simulink model "test_direct"  (R2024a)
settings: Solver=VariableStepAuto  StartTime=0.0  StopTime=40  RelTol=1e-3
libraries: neural x733, simulink x4
(part 16 of 35)

== system test_direct/Function Fitting Neural Network2/Layer 4/Delays 1 ==
  "p{4}" : Inport  PortDimensions=20
      mask Display: e = 0.06;c1 = [120 230 180]/255;c2 = ([120 230 180]+0)/(256+128);c3 = ([120 230 180]+128)/(256+128);patch([0 1 1 0],[0 0 1 1],c1);patch([0 1 1 1-e 1-e 0+e],[0 0 1 1-e 0+e 0+e],c2);patch([0 0 1 1-e 0+e 0+e],[0 1 1 1-e 1-e 0+e],c3);plot([0 1 1 0 0],[0 0 1 1 0]);
  mux : Mux  Inputs=1
      mask Display: e = 0.06;c1 = [120 150 230]/255;c2 = ([120 150 230]+0)/383;c3 = ([120 150 230]+128)/383;patch([0 1 1 0],[0 0 1 1],c1);patch([0 1 1 1-e 1-e 0+e],[0 0 1 1-e 0+e 0+e],c2);patch([0 0 1 1-e 0+e 0+e],[0 1 1 1-e 1-e 0+e],c3);plot([0 1 1 0 0],[0 0 1 1 0]);disp('Mux')
  "pd{4,3}" : Outport
      mask Display: e = 0.06;c1 = [120 230 180]/255;c2 = ([120 230 180]+0)/(256+128);c3 = ([120 230 180]+128)/(256+128);patch([0 1 1 0],[0 0 1 1],c1);patch([0 1 1 1-e 1-e 0+e],[0 0 1 1-e 0+e 0+e],c2);patch([0 0 1 1-e 0+e 0+e],[0 1 1 1-e 1-e 0+e],c3);plot([0 1 1 0 0],[0 0 1 1 0]);
  wires:
  "p{4}"/1 -> mux/1
  mux/1 -> "pd{4,3}"/1

== system test_direct/Function Fitting Neural Network2/Layer 4/LW{4,3} ==
  "ad{4,3}" : Inport  PortDimensions=20
      mask Display: e = 0.06;c1 = [120 230 180]/255;c2 = ([120 230 180]+0)/(256+128);c3 = ([120 230 180]+128)/(256+128);patch([0 1 1 0],[0 0 1 1],c1);patch([0 1 1 1-e 1-e 0+e],[0 0 1 1-e 0+e 0+e],c2);patch([0 0 1 1-e 0+e 0+e],[0 1 1 1-e 1-e 0+e],c3);plot([0 1 1 0 0],[0 0 1 1 0]);
  "IW{4,3}(1,:)'" : Constant  Value=[0.47244748817045678634940486517734825611114501953125;0.1834479136632027607145545289313304238021373748779296875;0.50676050579155818009979839189327321946620941162109375;-0.319327133366968662908647047515842132270336151123046875;0.381766967450572980435907766150194220244884490966796875;0.4563690535882181098514820405398495495319366455078125;0.198247183159460271806295850183232687413692474365234375;-0.33336007021097657787578327770461328327655792236328125;-0.412713567221942578822080349709722213447093963623046875;0.450498773156788934191041562371538020670413970947265625;0.25918714352219252017306416746578179299831390380859375;0.410400201848454049269321330939419567584991455078125;0.5409615578128141866187661435105837881565093994140625;-0.1653232740233982200894757852438488043844699859619140625;-0.462903675222519073173543802113272249698638916015625;-0.291527346498789807771601090280455537140369415283203125;0.0824641426334296323563677333368104882538318634033203125;0.1511362276477953570097412239192635752260684967041015625;0.211910610504960905675631011035875417292118072509765625;0.2073592739845122323583126444646040908992290496826171875]
      mask Display: e = 0.06;c1 = [120 150 230]/255;c2 = ([120 150 230]+0)/383;c3 = ([120 150 230]+128)/383;patch([0 1 1 0],[0 0 1 1],c1);patch([0 1 1 1-e 1-e 0+e],[0 0 1 1-e 0+e 0+e],c2);patch([0 0 1 1-e 0+e 0+e],[0 1 1 1-e 1-e 0+e],c3);plot([0 1 1 0 0],[0 0 1 1 0]);disp('weights');
  "IW{4,3}(10,:)'" : Constant  Value=[0.62004982880781611687126542165060527622699737548828125;-0.1719950517254123789623321272301836870610713958740234375;-0.181893759276586075568360456600203178822994232177734375;-0.2349075039028051536948993316400446929037570953369140625;-0.2452130522313871463513379467258346267044544219970703125;0.53580241435795894489046986564062535762786865234375;0.1931726513438345171902454922019387595355510711669921875;0.416953523146994131653997328612604178488254547119140625;0.397838857842025495070714669054723344743251800537109375;0.507717044004438289306335718720220029354095458984375;-0.09416114315560132619342681437046849168837070465087890625;-0.041804193884274531978206823623622767627239227294921875;0.220907364886507029400064539004233665764331817626953125;-0.39379811215660531775739627846633084118366241455078125;0.022802943761242200348959840994211845099925994873046875;-0.1133939581571223043088281201562494970858097076416015625;-0.11496157101289783408759603844373486936092376708984375;0.43779622024544206926321976425242610275745391845703125;0.55289807234135668334573665561038069427013397216796875;-0.064019714526170112822711644184892065823078155517578125]
      mask Display: e = 0.06;c1 = [120 150 230]/255;c2 = ([120 150 230]+0)/383;c3 = ([120 150 230]+128)/383;patch([0 1 1 0],[0 0 1 1],c1);patch([0 1 1 1-e 1-e 0+e],[0 0 1 1-e 0+e 0+e],c2);patch([0 0 1 1-e 0+e 0+e],[0 1 1 1-e 1-e 0+e],c3);plot([0 1 1 0 0],[0 0 1 1 0]);disp('weights');
  "IW{4,3}(2,:)'" : Constant  Value=[-0.52999007124834929260970284303766675293445587158203125;0.25866553837085659584005270517081953585147857666015625;-0.480994413539897192055860841719550080597400665283203125;0.5206363297816836155362807403434999287128448486328125;-0.051047340005507368942971879732795059680938720703125;0.397809270661283853609546667939866892993450164794921875;0.3484531918175519660252348330686800181865692138671875;0.108374910894089293567077447733026929199695587158203125;-0.28461804870320717153475698069087229669094085693359375;0.39361667333479866126566548700793646275997161865234375;0.5237614091308453456719007590436376631259918212890625;-0.157341307151045384227217027728329412639141082763671875;0.2175219008468349812801534426398575305938720703125;-0.09173383416637879983479564316439791582524776458740234375;-0.57629988642295171263896236268919892609119415283203125;0.4459283104025819621796244973666034638881683349609375;0.2831475555888369743939847467117942869663238525390625;-0.342059279452377740238233627678710035979747772216796875;-0.17909678064247780415740862736129201948642730712890625;-0.1831357131080906530673502174977329559624195098876953125]
      mask Display: e = 0.06;c1 = [120 150 230]/255;c2 = ([120 150 230]+0)/383;c3 = ([120 150 230]+128)/383;patch([0 1 1 0],[0 0 1 1],c1);patch([0 1 1 1-e 1-e 0+e],[0 0 1 1-e 0+e 0+e],c2);patch([0 0 1 1-e 0+e 0+e],[0 1 1 1-e 1-e 0+e],c3);plot([0 1 1 0 0],[0 0 1 1 0]);disp('weights');
  "IW{4,3}(3,:)'" : Constant  Value=[0.427271557113994393528599857745575718581676483154296875;-0.2427281184362371779794642634442425332963466644287109375;0.375438812590348280906482614227570593357086181640625;0.1887302950483509267343151805107481777667999267578125;0.442888527891407146608315770208719186484813690185546875;-0.145704452211226131996824051384464837610721588134765625;0.19332090468647444847505312282009981572628021240234375;0.2171117569728686635954773009871132671833038330078125;-0.42483570338458431780992441417765803635120391845703125;0.416898792982427546238710647230618633329868316650390625;0.09328037965492620708918281025034957565367221832275390625;-0.297160611411257435943156224311678670346736907958984375;-0.222561662706281693235865759561420418322086334228515625;-0.63635994313177512982093730897759087383747100830078125;0.0920557715904673223850096519527141936123371124267578125;0.046618920974470602625050474898671382106840610504150390625;0.517752265816589396507652054424397647380828857421875;0.481589341247303848181360308444709517061710357666015625;0.50223095070663681394051991446758620440959930419921875;0.351524225397905787371399810581351630389690399169921875]
      mask Display: e = 0.06;c1 = [120 150 230]/255;c2 = ([120 150 230]+0)/383;c3 = ([120 150 230]+128)/383;patch([0 1 1 0],[0 0 1 1],c1);patch([0 1 1 1-e 1-e 0+e],[0 0 1 1-e 0+e 0+e],c2);patch([0 0 1 1-e 0+e 0+e],[0 1 1 1-e 1-e 0+e],c3);plot([0 1 1 0 0],[0 0 1 1 0]);disp('weights');
  "IW{4,3}(4,:)'" : Constant  Value=[-0.4272419811355068208769125703838653862476348876953125;-0.218328695116062287961966603688779287040233612060546875;-0.267850284719499065477776866828207857906818389892578125;0.06203137737339370350042599966400302946567535400390625;-0.55900733287565085305459433584474027156829833984375;0.2032377842318154603784563505541882477700710296630859375;-0.20301371483371821735630646799108944833278656005859375;0.2093600985184538298966572256176732480525970458984375;0.35642519122358684580120780083234421908855438232421875;-0.449654061964883833280026692591491155326366424560546875;-0.39742954838629085401180418557487428188323974609375;-0.376347479489261782514830656509730033576488494873046875;0.10974448386632405794127720355390920303761959075927734375;0.341992937278279451884799300387385301291942596435546875;0.422196331780901046304421697641373611986637115478515625;0.3298742516092314502884619287215173244476318359375;0.3378712155354772761484127840958535671234130859375;0.20815576754154696548226866070763207972049713134765625;0.357266630131023277261448356512119062244892120361328125;-0.344625803699752264463995743426494300365447998046875]
      mask Display: e = 0.06;c1 = [120 150 230]/255;c2 = ([120 150 230]+0)/383;c3 = ([120 150 230]+128)/383;patch([0 1 1 0],[0 0 1 1],c1);patch([0 1 1 1-e 1-e 0+e],[0 0 1 1-e 0+e 0+e],c2);patch([0 0 1 1-e 0+e 0+e],[0 1 1 1-e 1-e 0+e],c3);plot([0 1 1 0 0],[0 0 1 1 0]);disp('weights');
  "IW{4,3}(5,:)'" : Constant  Value=[0.242125074488241442960401172967976890504360198974609375;-0.60473759647022851115849562120274640619754791259765625;0.404473610734588817638979207913507707417011260986328125;-0.2590760492587571572897786609246395528316497802734375;0.1405439339409519095003275879207649268209934234619140625;0.142911761057261277318986003592726774513721466064453125;0.351091239707742974740511954223620705306529998779296875;0.0960644091923418541600909748012782074511051177978515625;-0.45544304543415237152004237941582687199115753173828125;-0.60626839080967542816580362341483123600482940673828125;0.42183625826601645059099610080011188983917236328125;-0.386967076793109321375396802977775223553180694580078125;-0.340070110055025021100760795889073051512241363525390625;0.1002300444043862370779862658309866674244403839111328125;-0.10990293007616182274777116845143609680235385894775390625;0.55207704769645282727452695326064713299274444580078125;-0.31459192782915545993915884537273086607456207275390625;0.345382987134464414236134643942932598292827606201171875;0.249144363683819924926154953936929814517498016357421875;0.168080126592327683265892801500740461051464080810546875]
      mask Display: e = 0.06;c1 = [120 150 230]/255;c2 = ([120 150 230]+0)/383;c3 = ([120 150 230]+128)/383;patch([0 1 1 0],[0 0 1 1],c1);patch([0 1 1 1-e 1-e 0+e],[0 0 1 1-e 0+e 0+e],c2);patch([0 0 1 1-e 0+e 0+e],[0 1 1 1-e 1-e 0+e],c3);plot([0 1 1 0 0],[0 0 1 1 0]);disp('weights');
  "IW{4,3}(6,:)'" : Constant  Value=[0.436176279970378499850625075850985012948513031005859375;-0.451489036951920663653936571790836751461029052734375;0.08911938882860499788751695859900792129337787628173828125;-0.485863711992422453445072960676043294370174407958984375;0.127572397355813327290974257266498170793056488037109375;-0.63812853495278332172091495522181503474712371826171875;0.2818837491960926033840451054857112467288970947265625;-0.0131968716074592172515789201270308694802224636077880859375;0.1537834832577880395110270228542503900825977325439453125;0.48011264273196319063430337337194941937923431396484375;-0.207405778126915352199688413747935555875301361083984375;-0.09951366702140125586328878171116230078041553497314453125;-0.268246262611988417479125246245530433952808380126953125;-0.406874531488279178592648577250656671822071075439453125;0.03159486549302327473842666449854732491075992584228515625;0.30773203396346981985942647952469997107982635498046875;0.033399545565028616878056055838897009380161762237548828125;-0.101874376296882063197557499734102748334407806396484375;0.048492904628586297466341648032539524137973785400390625;-0.34122312837322377188087330068810842931270599365234375]
      mask Display: e = 0.06;c1 = [120 150 230]/255;c2 = ([120 150 230]+0)/383;c3 = ([120 150 230]+128)/383;patch([0 1 1 0],[0 0 1 1],c1);patch([0 1 1 1-e 1-e 0+e],[0 0 1 1-e 0+e 0+e],c2);patch([0 0 1 1-e 0+e 0+e],[0 1 1 1-e 1-e 0+e],c3);plot([0 1 1 0 0],[0 0 1 1 0]);disp('weights');
  "IW{4,3}(7,:)'" : Constant  Value=[-0.283546119620839309760640389868058264255523681640625;-0.10361342455437162757281299718670197762548923492431640625;-0.058161527580973100548522580766075407154858112335205078125;0.51121075013165506728540776748559437692165374755859375;0.29651416162894383976578183137462474405765533447265625;-0.1252198113694278358565270536928437650203704833984375;-0.157886646248348305743292030456359498202800750732421875;0.32110978088458230761403910946683026850223541259765625;0.308480031707026258747106339797028340399265289306640625;0.033278433162800026556826793466825620271265506744384765625;0.396616284348000502912867659688345156610012054443359375;0.34965408898041838714476625682436861097812652587890625;0.326379064754532766112760100440937094390392303466796875;-0.26442051443391767495683097877190448343753814697265625;-0.325375298162383697064825582856428809463977813720703125;-0.17882765495459873594796817997121252119541168212890625;0.6391344025452669885822842843481339514255523681640625;0.66604526975968758595314511694596149027347564697265625;-0.5674698696229978356342371625942178070545196533203125;-0.0895385469065017314260757075317087583243846893310546875]
      mask Display: e = 0.06;c1 = [120 150 230]/255;c2 = ([120 150 230]+0)/383;c3 = ([120 150 230]+128)/383;patch([0 1 1 0],[0 0 1 1],c1);patch([0 1 1 1-e 1-e 0+e],[0 0 1 1-e 0+e 0+e],c2);patch([0 0 1 1-e 0+e 0+e],[0 1 1 1-e 1-e 0+e],c3);plot([0 1 1 0 0],[0 0 1 1 0]);disp('weights');
  "IW{4,3}(8,:)'" : Constant  Value=[-0.44158180291790649629746212667669169604778289794921875;-0.29737887161936871205369925519335083663463592529296875;-0.1731668100134340360085616339347325265407562255859375;-0.189524413062696350795732769256574101746082305908203125;-0.1682336544676640566198244641782366670668125152587890625;-0.63990017329392590017533848367747850716114044189453125;-0.12091324308068292225915030257965554483234882354736328125;-0.08116268648245718309031104809037060476839542388916015625;-0.1777960634037018816666630982581409625709056854248046875;-0.16733851128191801205247202233294956386089324951171875;0.489923677023728687540682358303456567227840423583984375;0.369528344926653040669606298251892440021038055419921875;-0.268289530246816509961860219846130348742008209228515625;-0.287624994977375647575712491743615828454494476318359375;0.17883429478338219720257029621279798448085784912109375;-0.48206985790917233902774796661105938255786895751953125;-0.009881485170639754678223454220642452128231525421142578125;0.448369826626772771671625150702311657369136810302734375;0.6902728087614977692254569774377159774303436279296875;0.354051711308562111479858458551461808383464813232421875]
      mask Display: e = 0.06;c1 = [120 150 230]/255;c2 = ([120 150 230]+0)/383;c3 = ([120 150 230]+128)/383;patch([0 1 1 0],[0 0 1 1],c1);patch([0 1 1 1-e 1-e 0+e],[0 0 1 1-e 0+e 0+e],c2);patch([0 0 1 1-e 0+e 0+e],[0 1 1 1-e 1-e 0+e],c3);plot([0 1 1 0 0],[0 0 1 1 0]);disp('weights');
  "IW{4,3}(9,:)'" : Constant  Value=[-0.471070051569210723751979230655706487596035003662109375;0.00431051595087869783562428693812762503512203693389892578125;-0.1575641998254519726696543102661962620913982391357421875;-0.072561288605265616968864605951239354908466339111328125;-0.5805348839554176354482706301496364176273345947265625;0.379023161422289034394594864352256990969181060791015625;-0.456586292726742615233348487890907563269138336181640625;-0.17056625130829339287430457261507399380207061767578125;0.24047114638423916499476717945071868598461151123046875;-0.1748905466580590317704491098993457853794097900390625;0.050215249866397672351414627200938411988317966461181640625;0.238950903829427574454058458286453969776630401611328125;-0.11299356269503146865673670617979951202869415283203125;-0.59749277719319981994061663499451242387294769287109375;-0.382383860884375759159325980363064445555210113525390625;-0.58043042099357389229652426365646533668041229248046875;-0.05488111243213793233319819364623981527984142303466796875;-0.49967492911579303171976107478258199989795684814453125;0.40333471589349245700617530019371770322322845458984375;0.31340698801696564856911209062673151493072509765625]
      mask Display: e = 0.06;c1 = [120 150 230]/255;c2 = ([120 150 230]+0)/383;c3 = ([120 150 230]+128)/383;patch([0 1 1 0],[0 0 1 1],c1);patch([0 1 1 1-e 1-e 0+e],[0 0 1 1-e 0+e 0+e],c2);patch([0 0 1 1-e 0+e 0+e],[0 1 1 1-e 1-e 0+e],c3);plot([0 1 1 0 0],[0 0 1 1 0]);disp('weights');
  Mux : Mux  Inputs=10
      mask Display: e = 0.06;c1 = [120 150 230]/255;c2 = ([120 150 230]+0)/383;c3 = ([120 150 230]+128)/383;patch([0 1 1 0],[0 0 1 1],c1);patch([0 1 1 1-e 1-e 0+e],[0 0 1 1-e 0+e 0+e],c2);patch([0 0 1 1-e 0+e 0+e],[0 1 1 1-e 1-e 0+e],c3);plot([0 1 1 0 0],[0 0 1 1 0]);disp('Mux');
  dotprod{1..10} (10 alike) : neural/Weight Functions/dotprod
  "lz{4,3}" : Outport
      mask Display: e = 0.06;c1 = [120 230 180]/255;c2 = ([120 230 180]+0)/(256+128);c3 = ([120 230 180]+128)/(256+128);patch([0 1 1 0],[0 0 1 1],c1);patch([0 1 1 1-e 1-e 0+e],[0 0 1 1-e 0+e 0+e],c2);patch([0 0 1 1-e 0+e 0+e],[0 1 1 1-e 1-e 0+e],c3);plot([0 1 1 0 0],[0 0 1 1 0]);
  wires:
  "IW{4,3}(1,:)'"/1 -> dotprod1/1
  "ad{4,3}"/1 -> dotprod1/2, dotprod2/2, dotprod3/2, dotprod4/2, dotprod5/2, dotprod6/2, dotprod7/2, dotprod8/2, dotprod9/2, dotprod10/2
  dotprod1/1 -> Mux/1
  "IW{4,3}(2,:)'"/1 -> dotprod2/1
  dotprod2/1 -> Mux/2
  "IW{4,3}(3,:)'"/1 -> dotprod3/1
  dotprod3/1 -> Mux/3
  "IW{4,3}(4,:)'"/1 -> dotprod4/1
  dotprod4/1 -> Mux/4
  "IW{4,3}(5,:)'"/1 -> dotprod5/1
  dotprod5/1 -> Mux/5
  "IW{4,3}(6,:)'"/1 -> dotprod6/1
  dotprod6/1 -> Mux/6
  "IW{4,3}(7,:)'"/1 -> dotprod7/1
  dotprod7/1 -> Mux/7
  "IW{4,3}(8,:)'"/1 -> dotprod8/1
  dotprod8/1 -> Mux/8
  "IW{4,3}(9,:)'"/1 -> dotprod9/1
  dotprod9/1 -> Mux/9
  "IW{4,3}(10,:)'"/1 -> dotprod10/1
  dotprod10/1 -> Mux/10
  Mux/1 -> "lz{4,3}"/1

== system test_direct/Function Fitting Neural Network2/Layer 5/Delays 1 ==
  "p{5}" : Inport  PortDimensions=10
      mask Display: e = 0.06;c1 = [120 230 180]/255;c2 = ([120 230 180]+0)/(256+128);c3 = ([120 230 180]+128)/(256+128);patch([0 1 1 0],[0 0 1 1],c1);patch([0 1 1 1-e 1-e 0+e],[0 0 1 1-e 0+e 0+e],c2);patch([0 0 1 1-e 0+e 0+e],[0 1 1 1-e 1-e 0+e],c3);plot([0 1 1 0 0],[0 0 1 1 0]);
  mux : Mux  Inputs=1
      mask Display: e = 0.06;c1 = [120 150 230]/255;c2 = ([120 150 230]+0)/383;c3 = ([120 150 230]+128)/383;patch([0 1 1 0],[0 0 1 1],c1);patch([0 1 1 1-e 1-e 0+e],[0 0 1 1-e 0+e 0+e],c2);patch([0 0 1 1-e 0+e 0+e],[0 1 1 1-e 1-e 0+e],c3);plot([0 1 1 0 0],[0 0 1 1 0]);disp('Mux')
  "pd{5,4}" : Outport
      mask Display: e = 0.06;c1 = [120 230 180]/255;c2 = ([120 230 180]+0)/(256+128);c3 = ([120 230 180]+128)/(256+128);patch([0 1 1 0],[0 0 1 1],c1);patch([0 1 1 1-e 1-e 0+e],[0 0 1 1-e 0+e 0+e],c2);patch([0 0 1 1-e 0+e 0+e],[0 1 1 1-e 1-e 0+e],c3);plot([0 1 1 0 0],[0 0 1 1 0]);
  wires:
  "p{5}"/1 -> mux/1
  mux/1 -> "pd{5,4}"/1

== system test_direct/Function Fitting Neural Network2/Layer 5/LW{5,4} ==
  "ad{5,4}" : Inport  PortDimensions=10
      mask Display: e = 0.06;c1 = [120 230 180]/255;c2 = ([120 230 180]+0)/(256+128);c3 = ([120 230 180]+128)/(256+128);patch([0 1 1 0],[0 0 1 1],c1);patch([0 1 1 1-e 1-e 0+e],[0 0 1 1-e 0+e 0+e],c2);patch([0 0 1 1-e 0+e 0+e],[0 1 1 1-e 1-e 0+e],c3);plot([0 1 1 0 0],[0 0 1 1 0]);
  "IW{5,4}(1,:)'" : Constant  Value=[-0.67893230334680743087716336958692409098148345947265625;-0.7007735186931760562600857156212441623210906982421875;0.253289980978913031872679084699484519660472869873046875;-0.89589692731303116612906478621880523860454559326171875;-0.791589830532370086757509852759540081024169921875;-0.451582324523090161694227617772412486374378204345703125;-0.70110133568199817233335124910809099674224853515625;-0.92574724276718589610624121633009053766727447509765625;0.88375268226322234443870229370077140629291534423828125;0.52256981069607510992369725499884225428104400634765625]
      mask Display: e = 0.06;c1 = [120 150 230]/255;c2 = ([120 150 230]+0)/383;c3 = ([120 150 230]+128)/383;patch([0 1 1 0],[0 0 1 1],c1);patch([0 1 1 1-e 1-e 0+e],[0 0 1 1-e 0+e 0+e],c2);patch([0 0 1 1-e 0+e 0+e],[0 1 1 1-e 1-e 0+e],c3);plot([0 1 1 0 0],[0 0 1 1 0]);disp('weights');
  "IW{5,4}(2,:)'" : Constant  Value=[-0.785927457994070710611822505597956478595733642578125;0.809549628935909648674851268879137933254241943359375;0.320823297951406571915100585101754404604434967041015625;-0.6460974169776598774461717766826041042804718017578125;-0.5216632365400031279278891815920360386371612548828125;-0.60438186683382022490462759378715418279170989990234375;-0.318511865868724985961790707733598537743091583251953125;0.63479970676133412599284611133043654263019561767578125;-0.38058653289221933135877407039515674114227294921875;-0.7168981885025276223899481919943355023860931396484375]
      mask Display: e = 0.06;c1 = [120 150 230]/255;c2 = ([120 150 230]+0)/383;c3 = ([120 150 230]+128)/383;patch([0 1 1 0],[0 0 1 1],c1);patch([0 1 1 1-e 1-e 0+e],[0 0 1 1-e 0+e 0+e],c2);patch([0 0 1 1-e 0+e 0+e],[0 1 1 1-e 1-e 0+e],c3);plot([0 1 1 0 0],[0 0 1 1 0]);disp('weights');
  Mux : Mux  Inputs=2
      mask Display: e = 0.06;c1 = [120 150 230]/255;c2 = ([120 150 230]+0)/383;c3 = ([120 150 230]+128)/383;patch([0 1 1 0],[0 0 1 1],c1);patch([0 1 1 1-e 1-e 0+e],[0 0 1 1-e 0+e 0+e],c2);patch([0 0 1 1-e 0+e 0+e],[0 1 1 1-e 1-e 0+e],c3);plot([0 1 1 0 0],[0 0 1 1 0]);disp('Mux');
  dotprod1 : neural/Weight Functions/dotprod
  dotprod2 : neural/Weight Functions/dotprod
  "lz{5,4}" : Outport
      mask Display: e = 0.06;c1 = [120 230 180]/255;c2 = ([120 230 180]+0)/(256+128);c3 = ([120 230 180]+128)/(256+128);patch([0 1 1 0],[0 0 1 1],c1);patch([0 1 1 1-e 1-e 0+e],[0 0 1 1-e 0+e 0+e],c2);patch([0 0 1 1-e 0+e 0+e],[0 1 1 1-e 1-e 0+e],c3);plot([0 1 1 0 0],[0 0 1 1 0]);
  wires:
  "IW{5,4}(1,:)'"/1 -> dotprod1/1
  "ad{5,4}"/1 -> dotprod1/2, dotprod2/2
  dotprod1/1 -> Mux/1
  "IW{5,4}(2,:)'"/1 -> dotprod2/1
  dotprod2/1 -> Mux/2
  Mux/1 -> "lz{5,4}"/1

== system test_direct/Function Fitting Neural Network3/Layer 1/Delays 1 ==
  "p{1}" : Inport  PortDimensions=8
      mask Display: e = 0.06;c1 = [120 230 180]/255;c2 = ([120 230 180]+0)/(256+128);c3 = ([120 230 180]+128)/(256+128);patch([0 1 1 0],[0 0 1 1],c1);patch([0 1 1 1-e 1-e 0+e],[0 0 1 1-e 0+e 0+e],c2);patch([0 0 1 1-e 0+e 0+e],[0 1 1 1-e 1-e 0+e],c3);plot([0 1 1 0 0],[0 0 1 1 0]);
  mux : Mux  Inputs=1
      mask Display: e = 0.06;c1 = [120 150 230]/255;c2 = ([120 150 230]+0)/383;c3 = ([120 150 230]+128)/383;patch([0 1 1 0],[0 0 1 1],c1);patch([0 1 1 1-e 1-e 0+e],[0 0 1 1-e 0+e 0+e],c2);patch([0 0 1 1-e 0+e 0+e],[0 1 1 1-e 1-e 0+e],c3);plot([0 1 1 0 0],[0 0 1 1 0]);disp('Mux')
  "pd{1,1}" : Outport
      mask Display: e = 0.06;c1 = [120 230 180]/255;c2 = ([120 230 180]+0)/(256+128);c3 = ([120 230 180]+128)/(256+128);patch([0 1 1 0],[0 0 1 1],c1);patch([0 1 1 1-e 1-e 0+e],[0 0 1 1-e 0+e 0+e],c2);patch([0 0 1 1-e 0+e 0+e],[0 1 1 1-e 1-e 0+e],c3);plot([0 1 1 0 0],[0 0 1 1 0]);
  wires:
  "p{1}"/1 -> mux/1
  mux/1 -> "pd{1,1}"/1

== system test_direct/Function Fitting Neural Network3/Layer 1/IW{1,1} ==
  "pd{1,1}" : Inport  PortDimensions=8
      mask Display: e = 0.06;c1 = [120 230 180]/255;c2 = ([120 230 180]+0)/(256+128);c3 = ([120 230 180]+128)/(256+128);patch([0 1 1 0],[0 0 1 1],c1);patch([0 1 1 1-e 1-e 0+e],[0 0 1 1-e 0+e 0+e],c2);patch([0 0 1 1-e 0+e 0+e],[0 1 1 1-e 1-e 0+e],c3);plot([0 1 1 0 0],[0 0 1 1 0]);
  "IW{1,1}(1,:)'" : Constant  Value=[0.0892796833873695516725632614907226525247097015380859375;0.0487006269441907779782496845655259676277637481689453125;-1.0170897656269961562003345534321852028369903564453125;1.37446005126252490669003236689604818820953369140625;-1.16221244258872413723793215467594563961029052734375;-0.1661060361968494103468430012071621604263782501220703125;0.74082225028830539503843510829028673470020294189453125;-0.401225825184216844387918854408781044185161590576171875]
      mask Display: e = 0.06;c1 = [120 150 230]/255;c2 = ([120 150 230]+0)/383;c3 = ([120 150 230]+128)/383;patch([0 1 1 0],[0 0 1 1],c1);patch([0 1 1 1-e 1-e 0+e],[0 0 1 1-e 0+e 0+e],c2);patch([0 0 1 1-e 0+e 0+e],[0 1 1 1-e 1-e 0+e],c3);plot([0 1 1 0 0],[0 0 1 1 0]);disp('Weights');
  "IW{1,1}(10,:)'" : Constant  Value=[0.01303207869853410805216498147274251095950603485107421875;-0.04108451234308641009107532227062620222568511962890625;-0.9206795098713376201970959300524555146694183349609375;-1.0015969990095758834769412715104408562183380126953125;-0.60196618905606469329683250180096365511417388916015625;1.9909917063525035541005081540788523852825164794921875;0.534545004232178211367454423452727496623992919921875;0.0161492691731847486102946476194119895808398723602294921875]
      mask Display: e = 0.06;c1 = [120 150 230]/255;c2 = ([120 150 230]+0)/383;c3 = ([120 150 230]+128)/383;patch([0 1 1 0],[0 0 1 1],c1);patch([0 1 1 1-e 1-e 0+e],[0 0 1 1-e 0+e 0+e],c2);patch([0 0 1 1-e 0+e 0+e],[0 1 1 1-e 1-e 0+e],c3);plot([0 1 1 0 0],[0 0 1 1 0]);disp('Weights');
  "IW{1,1}(11,:)'" : Constant  Value=[0.0229711768377898473136866641652886755764484405517578125;-0.01034982700172441989761029645933376741595566272735595703125;0.0848641314624297427027244111741310916841030120849609375;1.0344003083349815330649335010093636810779571533203125;-0.7673332478128795930416572446119971573352813720703125;-0.450238633583883329780661597396829165518283843994140625;0.7942436411547049157633182403515093028545379638671875;1.4541634733156703074286042465246282517910003662109375]
      mask Display: e = 0.06;c1 = [120 150 230]/255;c2 = ([120 150 230]+0)/383;c3 = ([120 150 230]+128)/383;patch([0 1 1 0],[0 0 1 1],c1);patch([0 1 1 1-e 1-e 0+e],[0 0 1 1-e 0+e 0+e],c2);patch([0 0 1 1-e 0+e 0+e],[0 1 1 1-e 1-e 0+e],c3);plot([0 1 1 0 0],[0 0 1 1 0]);disp('Weights');
  "IW{1,1}(12,:)'" : Constant  Value=[-0.009907297114269915383477638215481420047581195831298828125;0.0196834325736417424523860830731791793368756771087646484375;0.27996426375517791118596733213053084909915924072265625;0.68801923190866010049404621895519085228443145751953125;0.89450386379519686297356884097098372876644134521484375;0.82521185256858065049101469412562437355518341064453125;-0.99190079953903109721835562595515511929988861083984375;-0.5177426509118523423325086696422658860683441162109375]
      mask Display: e = 0.06;c1 = [120 150 230]/255;c2 = ([120 150 230]+0)/383;c3 = ([120 150 230]+128)/383;patch([0 1 1 0],[0 0 1 1],c1);patch([0 1 1 1-e 1-e 0+e],[0 0 1 1-e 0+e 0+e],c2);patch([0 0 1 1-e 0+e 0+e],[0 1 1 1-e 1-e 0+e],c3);plot([0 1 1 0 0],[0 0 1 1 0]);disp('Weights');
  "IW{1,1}(13,:)'" : Constant  Value=[-0.228653458329835024276377453134045936167240142822265625;-0.1219684121520599739962875673882081173360347747802734375;-0.564819454133386411598394261091016232967376708984375;0.78736630116910699683785423985682427883148193359375;0.1674897651902171047400003089933306910097599029541015625;0.2040752196158785725099704677631962113082408905029296875;-0.181579968016822246301700261028599925339221954345703125;-0.400200470442380440427854182416922412812709808349609375]
      mask Display: e = 0.06;c1 = [120 150 230]/255;c2 = ([120 150 230]+0)/383;c3 = ([120 150 230]+128)/383;patch([0 1 1 0],[0 0 1 1],c1);patch([0 1 1 1-e 1-e 0+e],[0 0 1 1-e 0+e 0+e],c2);patch([0 0 1 1-e 0+e 0+e],[0 1 1 1-e 1-e 0+e],c3);plot([0 1 1 0 0],[0 0 1 1 0]);disp('Weights');
  "IW{1,1}(14,:)'" : Constant  Value=[-0.1324935102681321641426848145783878862857818603515625;-0.05183195894003396475557821077018161304295063018798828125;-0.333253473142711531540527403194573707878589630126953125;1.189089176648551404724685198743827641010284423828125;-0.2240230499533238661680201175840920768678188323974609375;-1.1707018441889964766033926935051567852497100830078125;0.4703065981801308748089240907575003802776336669921875;-0.0198133844122105849672177413367535336874425411224365234375]
      mask Display: e = 0.06;c1 = [120 150 230]/255;c2 = ([120 150 230]+0)/383;c3 = ([120 150 230]+128)/383;patch([0 1 1 0],[0 0 1 1],c1);patch([0 1 1 1-e 1-e 0+e],[0 0 1 1-e 0+e 0+e],c2);patch([0 0 1 1-e 0+e 0+e],[0 1 1 1-e 1-e 0+e],c3);plot([0 1 1 0 0],[0 0 1 1 0]);disp('Weights');
  "IW{1,1}(15,:)'" : Constant  Value=[0.035406872816297098316429270425942377187311649322509765625;-0.020790779005280424218682355785858817398548126220703125;0.80471778188271347875826222661999054253101348876953125;0.097230604677444432137889407385955564677715301513671875;1.2506010931359250459848908576532267034053802490234375;0.1437824481417473432287579271360300481319427490234375;-1.2316972506650289975738132852711714804172515869140625;1.2414752899159944288243195842369459569454193115234375]
      mask Display: e = 0.06;c1 = [120 150 230]/255;c2 = ([120 150 230]+0)/383;c3 = ([120 150 230]+128)/383;patch([0 1 1 0],[0 0 1 1],c1);patch([0 1 1 1-e 1-e 0+e],[0 0 1 1-e 0+e 0+e],c2);patch([0 0 1 1-e 0+e 0+e],[0 1 1 1-e 1-e 0+e],c3);plot([0 1 1 0 0],[0 0 1 1 0]);disp('Weights');
  "IW{1,1}(16,:)'" : Constant  Value=[-0.1537599820517437099187674220956978388130664825439453125;0.475780947317519686823317215385031886398792266845703125;0.79291978152351838549094509289716370403766632080078125;0.87690394377613067877774710723315365612506866455078125;0.82770141369227323568935617004171945154666900634765625;-0.150954642202800359829240051112719811499118804931640625;-0.8348793438010140288696447896654717624187469482421875;0.16969106410959799990934016022947616875171661376953125]
      mask Display: e = 0.06;c1 = [120 150 230]/255;c2 = ([120 150 230]+0)/383;c3 = ([120 150 230]+128)/383;patch([0 1 1 0],[0 0 1 1],c1);patch([0 1 1 1-e 1-e 0+e],[0 0 1 1-e 0+e 0+e],c2);patch([0 0 1 1-e 0+e 0+e],[0 1 1 1-e 1-e 0+e],c3);plot([0 1 1 0 0],[0 0 1 1 0]);disp('Weights');
  "IW{1,1}(17,:)'" : Constant  Value=[0.005980149671435563106525190590900820097886025905609130859375;0.00099885036304448349304963006289881377597339451313018798828125;-0.1105512166217759995046066023860475979745388031005859375;-0.8179090100863908308070904240594245493412017822265625;0.09255529269132158065591653439696528948843479156494140625;-0.467053797344156029769379756544367410242557525634765625;-0.388378906453989480862531991078867577016353607177734375;0.20814539022041367299920011646463535726070404052734375]
      mask Display: e = 0.06;c1 = [120 150 230]/255;c2 = ([120 150 230]+0)/383;c3 = ([120 150 230]+128)/383;patch([0 1 1 0],[0 0 1 1],c1);patch([0 1 1 1-e 1-e 0+e],[0 0 1 1-e 0+e 0+e],c2);patch([0 0 1 1-e 0+e 0+e],[0 1 1 1-e 1-e 0+e],c3);plot([0 1 1 0 0],[0 0 1 1 0]);disp('Weights');
  "IW{1,1}(18,:)'" : Constant  Value=[-0.073595060434536507809610839103697799146175384521484375;-0.0091859102405284602521629011562254163436591625213623046875;-0.03801444904076613229282344263992854394018650054931640625;-0.6078885794226283056929105441668070852756500244140625;-1.3632814012436649253601217424147762358188629150390625;0.354356062084684009239055058060330338776111602783203125;0.77273209294521638668129526195116341114044189453125;-0.7437812380027402081594800620223395526409149169921875]
      mask Display: e = 0.06;c1 = [120 150 230]/255;c2 = ([120 150 230]+0)/383;c3 = ([120 150 230]+128)/383;patch([0 1 1 0],[0 0 1 1],c1);patch([0 1 1 1-e 1-e 0+e],[0 0 1 1-e 0+e 0+e],c2);patch([0 0 1 1-e 0+e 0+e],[0 1 1 1-e 1-e 0+e],c3);plot([0 1 1 0 0],[0 0 1 1 0]);disp('Weights');
  "IW{1,1}(19,:)'" : Constant  Value=[0.006600463185552522989152368637633117032237350940704345703125;-0.00851733409297182088304456470950754010118544101715087890625;0.34493964471005289507132829385227523744106292724609375;0.52148265894161849320909141169977374374866485595703125;-0.53846738729407805923443675055750645697116851806640625;1.13195277966592389162769904942251741886138916015625;0.839145201159271270086037475266493856906890869140625;-1.061312169550226780501134271617047488689422607421875]
      mask Display: e = 0.06;c1 = [120 150 230]/255;c2 = ([120 150 230]+0)/383;c3 = ([120 150 230]+128)/383;patch([0 1 1 0],[0 0 1 1],c1);patch([0 1 1 1-e 1-e 0+e],[0 0 1 1-e 0+e 0+e],c2);patch([0 0 1 1-e 0+e 0+e],[0 1 1 1-e 1-e 0+e],c3);plot([0 1 1 0 0],[0 0 1 1 0]);disp('Weights');
  "IW{1,1}(2,:)'" : Constant  Value=[0.01524981250965061659041754893451070529408752918243408203125;-0.0222295442983809453385557475257883197627961635589599609375;0.429092120174361546514063547874684445559978485107421875;-0.6949189441624457064250464100041426718235015869140625;0.290852515212432882751869556159363128244876861572265625;-0.76503105227094891915839980356395244598388671875;-0.1933037210077497292104453663341701030731201171875;1.6992745627848024891903833122341893613338470458984375]
      mask Display: e = 0.06;c1 = [120 150 230]/255;c2 = ([120 150 230]+0)/383;c3 = ([120 150 230]+128)/383;patch([0 1 1 0],[0 0 1 1],c1);patch([0 1 1 1-e 1-e 0+e],[0 0 1 1-e 0+e 0+e],c2);patch([0 0 1 1-e 0+e 0+e],[0 1 1 1-e 1-e 0+e],c3);plot([0 1 1 0 0],[0 0 1 1 0]);disp('Weights');
  "IW{1,1}(20,:)'" : Constant  Value=[0.57509537924807807574012485929415561258792877197265625;0.0833381949143732481122270883133751340210437774658203125;1.1358737018700415521976765376166440546512603759765625;-0.6514073179089161502730576103203929960727691650390625;-0.55448550462321277709776268238783814013004302978515625;0.85376389335350533205115652890526689589023590087890625;-0.262060920606275171707011395483277738094329833984375;-0.53353886420796337031191569622023962438106536865234375]
      mask Display: e = 0.06;c1 = [120 150 230]/255;c2 = ([120 150 230]+0)/383;c3 = ([120 150 230]+128)/383;patch([0 1 1 0],[0 0 1 1],c1);patch([0 1 1 1-e 1-e 0+e],[0 0 1 1-e 0+e 0+e],c2);patch([0 0 1 1-e 0+e 0+e],[0 1 1 1-e 1-e 0+e],c3);plot([0 1 1 0 0],[0 0 1 1 0]);disp('Weights');
  "IW{1,1}(3,:)'" : Constant  Value=[0.052591725210979267668420789050287567079067230224609375;-0.1945658957336089123213440643667127005755901336669921875;0.96149035365177326628582932244171388447284698486328125;0.31973085447596705233053171468782238662242889404296875;-0.1059391304337825856496380083626718260347843170166015625;-0.999482535308938935258993296884000301361083984375;-0.0473618749756202495060364299206412397325038909912109375;0.383872061888702542642448634069296531379222869873046875]
      mask Display: e = 0.06;c1 = [120 150 230]/255;c2 = ([120 150 230]+0)/383;c3 = ([120 150 230]+128)/383;patch([0 1 1 0],[0 0 1 1],c1);patch([0 1 1 1-e 1-e 0+e],[0 0 1 1-e 0+e 0+e],c2);patch([0 0 1 1-e 0+e 0+e],[0 1 1 1-e 1-e 0+e],c3);plot([0 1 1 0 0],[0 0 1 1 0]);disp('Weights');
  "IW{1,1}(4,:)'" : Constant  Value=[0.08161511214763157717744235242207651026546955108642578125;0.0182174991765660619635891492862356244586408138275146484375;-0.315286045684413540612922588479705154895782470703125;0.189294495415870012156034363215439952909946441650390625;0.65133712311208602496748198973364196717739105224609375;1.0963005209689009600282361134304665029048919677734375;-0.14040159716066968886849508635350503027439117431640625;-1.2298411035623224574209189086104743182659149169921875]
      mask Display: e = 0.06;c1 = [120 150 230]/255;c2 = ([120 150 230]+0)/383;c3 = ([120 150 230]+128)/383;patch([0 1 1 0],[0 0 1 1],c1);patch([0 1 1 1-e 1-e 0+e],[0 0 1 1-e 0+e 0+e],c2);patch([0 0 1 1-e 0+e 0+e],[0 1 1 1-e 1-e 0+e],c3);plot([0 1 1 0 0],[0 0 1 1 0]);disp('Weights');
  "IW{1,1}(5,:)'" : Constant  Value=[-0.0935598547428390381330842728857533074915409088134765625;-0.0033382741010287209949825015797841842868365347385406494140625;0.544344038234270133358450038940645754337310791015625;0.51819454095816153138542858869186602532863616943359375;-0.5899132457038016585926243351423181593418121337890625;-0.60676138067934803910219443423557095229625701904296875;0.77657040227627993633774394766078330576419830322265625;0.81263783516915377713729640163364820182323455810546875]
      mask Display: e = 0.06;c1 = [120 150 230]/255;c2 = ([120 150 230]+0)/383;c3 = ([120 150 230]+128)/383;patch([0 1 1 0],[0 0 1 1],c1);patch([0 1 1 1-e 1-e 0+e],[0 0 1 1-e 0+e 0+e],c2);patch([0 0 1 1-e 0+e 0+e],[0 1 1 1-e 1-e 0+e],c3);plot([0 1 1 0 0],[0 0 1 1 0]);disp('Weights');
  "IW{1,1}(6,:)'" : Constant  Value=[-0.00975974606563877015996677499742872896604239940643310546875;-0.0167523889131338081515121274378543603233993053436279296875;0.265384601690886900993149311034358106553554534912109375;0.7900465855269354076284571419819258153438568115234375;-0.46098990490868974045923778248834423720836639404296875;-0.01150829307690741203085149635398920509032905101776123046875;-0.0211368854382073569075917163218036876060068607330322265625;0.305165268076589446533120053572929464280605316162109375]
      mask Display: e = 0.06;c1 = [120 150 230]/255;c2 = ([120 150 230]+0)/383;c3 = ([120 150 230]+128)/383;patch([0 1 1 0],[0 0 1 1],c1);patch([0 1 1 1-e 1-e 0+e],[0 0 1 1-e 0+e 0+e],c2);patch([0 0 1 1-e 0+e 0+e],[0 1 1 1-e 1-e 0+e],c3);plot([0 1 1 0 0],[0 0 1 1 0]);disp('Weights');
  "IW{1,1}(7,:)'" : Constant  Value=[0.0038307670043931664992375996092732748365961015224456787109375;-0.01398990532168104504451289216149234562180936336517333984375;-0.54564970498991016700784939530421979725360870361328125;-0.162726789977850450075180788189754821360111236572265625;1.311800988815063906400837367982603609561920166015625;-0.2455310210887416688674278475446044467389583587646484375;-1.1330680417885481414685955314780585467815399169921875;0.9892059839311337920975120141520164906978607177734375]
      mask Display: e = 0.06;c1 = [120 150 230]/255;c2 = ([120 150 230]+0)/383;c3 = ([120 150 230]+128)/383;patch([0 1 1 0],[0 0 1 1],c1);patch([0 1 1 1-e 1-e 0+e],[0 0 1 1-e 0+e 0+e],c2);patch([0 0 1 1-e 0+e 0+e],[0 1 1 1-e 1-e 0+e],c3);plot([0 1 1 0 0],[0 0 1 1 0]);disp('Weights');
  "IW{1,1}(8,:)'" : Constant  Value=[0.0127287802029154295535562368968385271728038787841796875;0.0010849309841137176092795701976001510047353804111480712890625;0.649541129693549823542753074434585869312286376953125;-0.463961913447071994109904835568158887326717376708984375;0.782761427876142779069823518511839210987091064453125;0.29751843903156383053243416725308634340763092041015625;-0.266583128683179959583782192567014135420322418212890625;0.91507830978956572476334940802189521491527557373046875]
      mask Display: e = 0.06;c1 = [120 150 230]/255;c2 = ([120 150 230]+0)/383;c3 = ([120 150 230]+128)/383;patch([0 1 1 0],[0 0 1 1],c1);patch([0 1 1 1-e 1-e 0+e],[0 0 1 1-e 0+e 0+e],c2);patch([0 0 1 1-e 0+e 0+e],[0 1 1 1-e 1-e 0+e],c3);plot([0 1 1 0 0],[0 0 1 1 0]);disp('Weights');
  "IW{1,1}(9,:)'" : Constant  Value=[0.0196227321268475467241909626636697794310748577117919921875;-0.000794322881975736126182463525680077509605325758457183837890625;0.134669011175101493993366830181912519037723541259765625;-0.8073145630587761356622422681539319455623626708984375;0.08825635644900965692816185992342070676386356353759765625;0.164615478955909499969578746458864770829677581787109375;-0.471879572514027234575451075215823948383331298828125;-1.1661539218106791171436498188995756208896636962890625]
      mask Display: e = 0.06;c1 = [120 150 230]/255;c2 = ([120 150 230]+0)/383;c3 = ([120 150 230]+128)/383;patch([0 1 1 0],[0 0 1 1],c1);patch([0 1 1 1-e 1-e 0+e],[0 0 1 1-e 0+e 0+e],c2);patch([0 0 1 1-e 0+e 0+e],[0 1 1 1-e 1-e 0+e],c3);plot([0 1 1 0 0],[0 0 1 1 0]);disp('Weights');
  Mux : Mux  Inputs=20
      mask Display: e = 0.06;c1 = [120 150 230]/255;c2 = ([120 150 230]+0)/383;c3 = ([120 150 230]+128)/383;patch([0 1 1 0],[0 0 1 1],c1);patch([0 1 1 1-e 1-e 0+e],[0 0 1 1-e 0+e 0+e],c2);patch([0 0 1 1-e 0+e 0+e],[0 1 1 1-e 1-e 0+e],c3);plot([0 1 1 0 0],[0 0 1 1 0]);disp('Mux');
  dotprod{1..20} (20 alike) : neural/Weight Functions/dotprod
  "iz{1,1}" : Outport
      mask Display: e = 0.06;c1 = [120 230 180]/255;c2 = ([120 230 180]+0)/(256+128);c3 = ([120 230 180]+128)/(256+128);patch([0 1 1 0],[0 0 1 1],c1);patch([0 1 1 1-e 1-e 0+e],[0 0 1 1-e 0+e 0+e],c2);patch([0 0 1 1-e 0+e 0+e],[0 1 1 1-e 1-e 0+e],c3);plot([0 1 1 0 0],[0 0 1 1 0]);
  wires:
  "IW{1,1}(1,:)'"/1 -> dotprod1/1
  "pd{1,1}"/1 -> dotprod1/2, dotprod2/2, dotprod3/2, dotprod4/2, dotprod5/2, dotprod6/2, dotprod7/2, dotprod8/2, dotprod9/2, dotprod10/2, dotprod11/2, dotprod12/2, dotprod13/2, dotprod14/2, dotprod15/2, dotprod16/2, dotprod17/2, dotprod18/2, dotprod19/2, dotprod20/2
  dotprod1/1 -> Mux/1
  "IW{1,1}(2,:)'"/1 -> dotprod2/1
  dotprod2/1 -> Mux/2
  "IW{1,1}(3,:)'"/1 -> dotprod3/1
  dotprod3/1 -> Mux/3
  "IW{1,1}(4,:)'"/1 -> dotprod4/1
  dotprod4/1 -> Mux/4
  "IW{1,1}(5,:)'"/1 -> dotprod5/1
  dotprod5/1 -> Mux/5
  "IW{1,1}(6,:)'"/1 -> dotprod6/1
  dotprod6/1 -> Mux/6
  "IW{1,1}(7,:)'"/1 -> dotprod7/1
  dotprod7/1 -> Mux/7
  "IW{1,1}(8,:)'"/1 -> dotprod8/1
  dotprod8/1 -> Mux/8
  "IW{1,1}(9,:)'"/1 -> dotprod9/1
  dotprod9/1 -> Mux/9
  "IW{1,1}(10,:)'"/1 -> dotprod10/1
  dotprod10/1 -> Mux/10
  "IW{1,1}(11,:)'"/1 -> dotprod11/1
  dotprod11/1 -> Mux/11
  "IW{1,1}(12,:)'"/1 -> dotprod12/1
  dotprod12/1 -> Mux/12
  "IW{1,1}(13,:)'"/1 -> dotprod13/1
  dotprod13/1 -> Mux/13
  "IW{1,1}(14,:)'"/1 -> dotprod14/1
  dotprod14/1 -> Mux/14
  "IW{1,1}(15,:)'"/1 -> dotprod15/1
  dotprod15/1 -> Mux/15
  "IW{1,1}(16,:)'"/1 -> dotprod16/1
  dotprod16/1 -> Mux/16
  "IW{1,1}(17,:)'"/1 -> dotprod17/1
  dotprod17/1 -> Mux/17
  "IW{1,1}(18,:)'"/1 -> dotprod18/1
  dotprod18/1 -> Mux/18
  "IW{1,1}(19,:)'"/1 -> dotprod19/1
  dotprod19/1 -> Mux/19
  "IW{1,1}(20,:)'"/1 -> dotprod20/1
  dotprod20/1 -> Mux/20
  Mux/1 -> "iz{1,1}"/1

== system test_direct/Function Fitting Neural Network3/Layer 2/Delays 1 ==
  "p{2}" : Inport  PortDimensions=20
      mask Display: e = 0.06;c1 = [120 230 180]/255;c2 = ([120 230 180]+0)/(256+128);c3 = ([120 230 180]+128)/(256+128);patch([0 1 1 0],[0 0 1 1],c1);patch([0 1 1 1-e 1-e 0+e],[0 0 1 1-e 0+e 0+e],c2);patch([0 0 1 1-e 0+e 0+e],[0 1 1 1-e 1-e 0+e],c3);plot([0 1 1 0 0],[0 0 1 1 0]);
  mux : Mux  Inputs=1
      mask Display: e = 0.06;c1 = [120 150 230]/255;c2 = ([120 150 230]+0)/383;c3 = ([120 150 230]+128)/383;patch([0 1 1 0],[0 0 1 1],c1);patch([0 1 1 1-e 1-e 0+e],[0 0 1 1-e 0+e 0+e],c2);patch([0 0 1 1-e 0+e 0+e],[0 1 1 1-e 1-e 0+e],c3);plot([0 1 1 0 0],[0 0 1 1 0]);disp('Mux')
  "pd{2,1}" : Outport
      mask Display: e = 0.06;c1 = [120 230 180]/255;c2 = ([120 230 180]+0)/(256+128);c3 = ([120 230 180]+128)/(256+128);patch([0 1 1 0],[0 0 1 1],c1);patch([0 1 1 1-e 1-e 0+e],[0 0 1 1-e 0+e 0+e],c2);patch([0 0 1 1-e 0+e 0+e],[0 1 1 1-e 1-e 0+e],c3);plot([0 1 1 0 0],[0 0 1 1 0]);
  wires:
  "p{2}"/1 -> mux/1
  mux/1 -> "pd{2,1}"/1
